simulink model "gm_soc_dvbs2_fpga"  (R2025b)
settings: Solver=VariableStepAuto  StartTime=0.0  StopTime=10.0  RelTol=1e-3
InitFcn:
  | soc_dvbs2_init;
undefined symbols (not defined in the file or in its folder): Add, coefficientsLog, coefficientsSqrt1, coefficientsSqrt2, dataBits, Deinterleaver, designMultirateFIR, noisePow, Shift, Short, soc_dvbs2_designFIRFilter, soc_dvbs2_txPacketBits, syncWord, txDataOut, txFiltCoeff, XData
libraries: simulink x304, hdlsllib x265, dspsigops x15, dsphdlfiltering2 x8, hdlmdlgenlib x6, dsphdlsigops2 x5, commseqgen3 x5, dsphdlmathfun2 x3, hwlogicconnlib x2, whdledac x2, commhdlcrc x2, whdlutilities x1
(part 33 of 36)

== system gm_soc_dvbs2_fpga/DVBS2/DVBS2 TxRx/DVB-S2 HDL Receiver/Synchronizer and PL Header Decoder/PL Header Recovery/PL Header Decoder/ML Decoder/Integer to Bit Convertor/For Each Subsystem6_instance5 ==
  note: For Each
  In1 : Inport  OutDataTypeStr=fixdt(0, 4, 0)  PortDimensions=1  SampleTime=2.5e-07
  Extract Bits2 : simulink/Logic and Bit Operations/Extract Bits  bitsToExtract=Upper half  numBits=8  bitIdxRange=[32 63]  outScalingMode=Treat bit field as an integer
  Extract Bits3 : simulink/Logic and Bit Operations/Extract Bits  bitsToExtract=Lower half  numBits=8  bitIdxRange=[32 63]  outScalingMode=Treat bit field as an integer
  Mux1 : Mux  Inputs=2
  Out1 : Outport  SampleTime=2.5e-07
  wires:
  In1/1 -> Extract Bits2/1, Extract Bits3/1
  Extract Bits3/1 -> Mux1/2
  Extract Bits2/1 -> Mux1/1
  Mux1/1 -> Out1/1

== system gm_soc_dvbs2_fpga/DVBS2/DVBS2 TxRx/DVB-S2 HDL Receiver/Synchronizer and PL Header Decoder/PL Header Recovery/PL Header Decoder/ML Decoder/Integer to Bit Convertor/For Each Subsystem6_instance6 ==
  note: For Each
  In1 : Inport  OutDataTypeStr=fixdt(0, 4, 0)  PortDimensions=1  SampleTime=2.5e-07
  Extract Bits2 : simulink/Logic and Bit Operations/Extract Bits  bitsToExtract=Upper half  numBits=8  bitIdxRange=[32 63]  outScalingMode=Treat bit field as an integer
  Extract Bits3 : simulink/Logic and Bit Operations/Extract Bits  bitsToExtract=Lower half  numBits=8  bitIdxRange=[32 63]  outScalingMode=Treat bit field as an integer
  Mux1 : Mux  Inputs=2
  Out1 : Outport  SampleTime=2.5e-07
  wires:
  Extract Bits3/1 -> Mux1/2
  In1/1 -> Extract Bits2/1, Extract Bits3/1
  Extract Bits2/1 -> Mux1/1
  Mux1/1 -> Out1/1

== system gm_soc_dvbs2_fpga/DVBS2/DVBS2 TxRx/DVB-S2 HDL Receiver/Synchronizer and PL Header Decoder/PL Header Recovery/PL Header Decoder/ML Decoder/Integer to Bit Convertor/For Each Subsystem6_instance7 ==
  note: For Each
  In1 : Inport  OutDataTypeStr=fixdt(0, 4, 0)  PortDimensions=1  SampleTime=2.5e-07
  Extract Bits2 : simulink/Logic and Bit Operations/Extract Bits  bitsToExtract=Upper half  numBits=8  bitIdxRange=[32 63]  outScalingMode=Treat bit field as an integer
  Extract Bits3 : simulink/Logic and Bit Operations/Extract Bits  bitsToExtract=Lower half  numBits=8  bitIdxRange=[32 63]  outScalingMode=Treat bit field as an integer
  Mux1 : Mux  Inputs=2
  Out1 : Outport  SampleTime=2.5e-07
  wires:
  In1/1 -> Extract Bits2/1, Extract Bits3/1
  Extract Bits3/1 -> Mux1/2
  Extract Bits2/1 -> Mux1/1
  Mux1/1 -> Out1/1

== system gm_soc_dvbs2_fpga/DVBS2/DVBS2 TxRx/DVB-S2 HDL Receiver/Synchronizer and PL Header Decoder/PL Header Recovery/PL Header Decoder/ML Decoder/Integer to Bit Convertor/For Each Subsystem6_instance8 ==
  note: For Each
  In1 : Inport  OutDataTypeStr=fixdt(0, 4, 0)  PortDimensions=1  SampleTime=2.5e-07
  Extract Bits2 : simulink/Logic and Bit Operations/Extract Bits  bitsToExtract=Upper half  numBits=8  bitIdxRange=[32 63]  outScalingMode=Treat bit field as an integer
  Extract Bits3 : simulink/Logic and Bit Operations/Extract Bits  bitsToExtract=Lower half  numBits=8  bitIdxRange=[32 63]  outScalingMode=Treat bit field as an integer
  Mux1 : Mux  Inputs=2
  Out1 : Outport  SampleTime=2.5e-07
  wires:
  In1/1 -> Extract Bits3/1, Extract Bits2/1
  Extract Bits2/1 -> Mux1/1
  Extract Bits3/1 -> Mux1/2
  Mux1/1 -> Out1/1

== system gm_soc_dvbs2_fpga/DVBS2/DVBS2 TxRx/DVB-S2 HDL Receiver/Synchronizer and PL Header Decoder/PL Header Recovery/PL Header Decoder/ML Decoder/Integer to Bit Convertor/For Each Subsystem7_instance1 ==
  note: For Each
  In1 : Inport  OutDataTypeStr=fixdt(0, 2, 0)  PortDimensions=1  SampleTime=2.5e-07
  Extract Bits2 : simulink/Logic and Bit Operations/Extract Bits  bitsToExtract=Upper half  numBits=8  bitIdxRange=[32 63]  outScalingMode=Treat bit field as an integer
  Extract Bits3 : simulink/Logic and Bit Operations/Extract Bits  bitsToExtract=Lower half  numBits=8  bitIdxRange=[32 63]  outScalingMode=Treat bit field as an integer
  Mux1 : Mux  Inputs=2
  Out1 : Outport  SampleTime=2.5e-07
  wires:
  Extract Bits3/1 -> Mux1/2
  In1/1 -> Extract Bits2/1, Extract Bits3/1
  Extract Bits2/1 -> Mux1/1
  Mux1/1 -> Out1/1

== system gm_soc_dvbs2_fpga/DVBS2/DVBS2 TxRx/DVB-S2 HDL Receiver/Synchronizer and PL Header Decoder/PL Header Recovery/PL Header Decoder/ML Decoder/Integer to Bit Convertor/For Each Subsystem7_instance10 ==
  note: For Each
  In1 : Inport  OutDataTypeStr=fixdt(0, 2, 0)  PortDimensions=1  SampleTime=2.5e-07
  Extract Bits2 : simulink/Logic and Bit Operations/Extract Bits  bitsToExtract=Upper half  numBits=8  bitIdxRange=[32 63]  outScalingMode=Treat bit field as an integer
  Extract Bits3 : simulink/Logic and Bit Operations/Extract Bits  bitsToExtract=Lower half  numBits=8  bitIdxRange=[32 63]  outScalingMode=Treat bit field as an integer
  Mux1 : Mux  Inputs=2
  Out1 : Outport  SampleTime=2.5e-07
  wires:
  In1/1 -> Extract Bits2/1, Extract Bits3/1
  Extract Bits3/1 -> Mux1/2
  Extract Bits2/1 -> Mux1/1
  Mux1/1 -> Out1/1

== system gm_soc_dvbs2_fpga/DVBS2/DVBS2 TxRx/DVB-S2 HDL Receiver/Synchronizer and PL Header Decoder/PL Header Recovery/PL Header Decoder/ML Decoder/Integer to Bit Convertor/For Each Subsystem7_instance11 ==
  note: For Each
  In1 : Inport  OutDataTypeStr=fixdt(0, 2, 0)  PortDimensions=1  SampleTime=2.5e-07
  Extract Bits2 : simulink/Logic and Bit Operations/Extract Bits  bitsToExtract=Upper half  numBits=8  bitIdxRange=[32 63]  outScalingMode=Treat bit field as an integer
  Extract Bits3 : simulink/Logic and Bit Operations/Extract Bits  bitsToExtract=Lower half  numBits=8  bitIdxRange=[32 63]  outScalingMode=Treat bit field as an integer
  Mux1 : Mux  Inputs=2
  Out1 : Outport  SampleTime=2.5e-07
  wires:
  In1/1 -> Extract Bits2/1, Extract Bits3/1
  Extract Bits2/1 -> Mux1/1
  Extract Bits3/1 -> Mux1/2
  Mux1/1 -> Out1/1

== system gm_soc_dvbs2_fpga/DVBS2/DVBS2 TxRx/DVB-S2 HDL Receiver/Synchronizer and PL Header Decoder/PL Header Recovery/PL Header Decoder/ML Decoder/Integer to Bit Convertor/For Each Subsystem7_instance12 ==
  note: For Each
  In1 : Inport  OutDataTypeStr=fixdt(0, 2, 0)  PortDimensions=1  SampleTime=2.5e-07
  Extract Bits2 : simulink/Logic and Bit Operations/Extract Bits  bitsToExtract=Upper half  numBits=8  bitIdxRange=[32 63]  outScalingMode=Treat bit field as an integer
  Extract Bits3 : simulink/Logic and Bit Operations/Extract Bits  bitsToExtract=Lower half  numBits=8  bitIdxRange=[32 63]  outScalingMode=Treat bit field as an integer
  Mux1 : Mux  Inputs=2
  Out1 : Outport  SampleTime=2.5e-07
  wires:
  Extract Bits3/1 -> Mux1/2
  In1/1 -> Extract Bits2/1, Extract Bits3/1
  Extract Bits2/1 -> Mux1/1
  Mux1/1 -> Out1/1

== system gm_soc_dvbs2_fpga/DVBS2/DVBS2 TxRx/DVB-S2 HDL Receiver/Synchronizer and PL Header Decoder/PL Header Recovery/PL Header Decoder/ML Decoder/Integer to Bit Convertor/For Each Subsystem7_instance13 ==
  note: For Each
  In1 : Inport  OutDataTypeStr=fixdt(0, 2, 0)  PortDimensions=1  SampleTime=2.5e-07
  Extract Bits2 : simulink/Logic and Bit Operations/Extract Bits  bitsToExtract=Upper half  numBits=8  bitIdxRange=[32 63]  outScalingMode=Treat bit field as an integer
  Extract Bits3 : simulink/Logic and Bit Operations/Extract Bits  bitsToExtract=Lower half  numBits=8  bitIdxRange=[32 63]  outScalingMode=Treat bit field as an integer
  Mux1 : Mux  Inputs=2
  Out1 : Outport  SampleTime=2.5e-07
  wires:
  In1/1 -> Extract Bits2/1, Extract Bits3/1
  Extract Bits3/1 -> Mux1/2
  Extract Bits2/1 -> Mux1/1
  Mux1/1 -> Out1/1

== system gm_soc_dvbs2_fpga/DVBS2/DVBS2 TxRx/DVB-S2 HDL Receiver/Synchronizer and PL Header Decoder/PL Header Recovery/PL Header Decoder/ML Decoder/Integer to Bit Convertor/For Each Subsystem7_instance14 ==
  note: For Each
  In1 : Inport  OutDataTypeStr=fixdt(0, 2, 0)  PortDimensions=1  SampleTime=2.5e-07
  Extract Bits2 : simulink/Logic and Bit Operations/Extract Bits  bitsToExtract=Upper half  numBits=8  bitIdxRange=[32 63]  outScalingMode=Treat bit field as an integer
  Extract Bits3 : simulink/Logic and Bit Operations/Extract Bits  bitsToExtract=Lower half  numBits=8  bitIdxRange=[32 63]  outScalingMode=Treat bit field as an integer
  Mux1 : Mux  Inputs=2
  Out1 : Outport  SampleTime=2.5e-07
  wires:
  Extract Bits3/1 -> Mux1/2
  In1/1 -> Extract Bits2/1, Extract Bits3/1
  Extract Bits2/1 -> Mux1/1
  Mux1/1 -> Out1/1

== system gm_soc_dvbs2_fpga/DVBS2/DVBS2 TxRx/DVB-S2 HDL Receiver/Synchronizer and PL Header Decoder/PL Header Recovery/PL Header Decoder/ML Decoder/Integer to Bit Convertor/For Each Subsystem7_instance15 ==
  note: For Each
  In1 : Inport  OutDataTypeStr=fixdt(0, 2, 0)  PortDimensions=1  SampleTime=2.5e-07
  Extract Bits2 : simulink/Logic and Bit Operations/Extract Bits  bitsToExtract=Upper half  numBits=8  bitIdxRange=[32 63]  outScalingMode=Treat bit field as an integer
  Extract Bits3 : simulink/Logic and Bit Operations/Extract Bits  bitsToExtract=Lower half  numBits=8  bitIdxRange=[32 63]  outScalingMode=Treat bit field as an integer
  Mux1 : Mux  Inputs=2
  Out1 : Outport  SampleTime=2.5e-07
  wires:
  In1/1 -> Extract Bits2/1, Extract Bits3/1
  Extract Bits3/1 -> Mux1/2
  Extract Bits2/1 -> Mux1/1
  Mux1/1 -> Out1/1

== system gm_soc_dvbs2_fpga/DVBS2/DVBS2 TxRx/DVB-S2 HDL Receiver/Synchronizer and PL Header Decoder/PL Header Recovery/PL Header Decoder/ML Decoder/Integer to Bit Convertor/For Each Subsystem7_instance16 ==
  note: For Each
  In1 : Inport  OutDataTypeStr=fixdt(0, 2, 0)  PortDimensions=1  SampleTime=2.5e-07
  Extract Bits2 : simulink/Logic and Bit Operations/Extract Bits  bitsToExtract=Upper half  numBits=8  bitIdxRange=[32 63]  outScalingMode=Treat bit field as an integer
  Extract Bits3 : simulink/Logic and Bit Operations/Extract Bits  bitsToExtract=Lower half  numBits=8  bitIdxRange=[32 63]  outScalingMode=Treat bit field as an integer
  Mux1 : Mux  Inputs=2
  Out1 : Outport  SampleTime=2.5e-07
  wires:
  Extract Bits3/1 -> Mux1/2
  In1/1 -> Extract Bits2/1, Extract Bits3/1
  Extract Bits2/1 -> Mux1/1
  Mux1/1 -> Out1/1

== system gm_soc_dvbs2_fpga/DVBS2/DVBS2 TxRx/DVB-S2 HDL Receiver/Synchronizer and PL Header Decoder/PL Header Recovery/PL Header Decoder/ML Decoder/Integer to Bit Convertor/For Each Subsystem7_instance2 ==
  note: For Each
  In1 : Inport  OutDataTypeStr=fixdt(0, 2, 0)  PortDimensions=1  SampleTime=2.5e-07
  Extract Bits2 : simulink/Logic and Bit Operations/Extract Bits  bitsToExtract=Upper half  numBits=8  bitIdxRange=[32 63]  outScalingMode=Treat bit field as an integer
  Extract Bits3 : simulink/Logic and Bit Operations/Extract Bits  bitsToExtract=Lower half  numBits=8  bitIdxRange=[32 63]  outScalingMode=Treat bit field as an integer
  Mux1 : Mux  Inputs=2
  Out1 : Outport  SampleTime=2.5e-07
  wires:
  Extract Bits3/1 -> Mux1/2
  In1/1 -> Extract Bits2/1, Extract Bits3/1
  Extract Bits2/1 -> Mux1/1
  Mux1/1 -> Out1/1

== system gm_soc_dvbs2_fpga/DVBS2/DVBS2 TxRx/DVB-S2 HDL Receiver/Synchronizer and PL Header Decoder/PL Header Recovery/PL Header Decoder/ML Decoder/Integer to Bit Convertor/For Each Subsystem7_instance3 ==
  note: For Each
  In1 : Inport  OutDataTypeStr=fixdt(0, 2, 0)  PortDimensions=1  SampleTime=2.5e-07
  Extract Bits2 : simulink/Logic and Bit Operations/Extract Bits  bitsToExtract=Upper half  numBits=8  bitIdxRange=[32 63]  outScalingMode=Treat bit field as an integer
  Extract Bits3 : simulink/Logic and Bit Operations/Extract Bits  bitsToExtract=Lower half  numBits=8  bitIdxRange=[32 63]  outScalingMode=Treat bit field as an integer
  Mux1 : Mux  Inputs=2
  Out1 : Outport  SampleTime=2.5e-07
  wires:
  In1/1 -> Extract Bits2/1, Extract Bits3/1
  Extract Bits3/1 -> Mux1/2
  Extract Bits2/1 -> Mux1/1
  Mux1/1 -> Out1/1

== system gm_soc_dvbs2_fpga/DVBS2/DVBS2 TxRx/DVB-S2 HDL Receiver/Synchronizer and PL Header Decoder/PL Header Recovery/PL Header Decoder/ML Decoder/Integer to Bit Convertor/For Each Subsystem7_instance4 ==
  note: For Each
  In1 : Inport  OutDataTypeStr=fixdt(0, 2, 0)  PortDimensions=1  SampleTime=2.5e-07
  Extract Bits2 : simulink/Logic and Bit Operations/Extract Bits  bitsToExtract=Upper half  numBits=8  bitIdxRange=[32 63]  outScalingMode=Treat bit field as an integer
  Extract Bits3 : simulink/Logic and Bit Operations/Extract Bits  bitsToExtract=Lower half  numBits=8  bitIdxRange=[32 63]  outScalingMode=Treat bit field as an integer
  Mux1 : Mux  Inputs=2
  Out1 : Outport  SampleTime=2.5e-07
  wires:
  Extract Bits3/1 -> Mux1/2
  In1/1 -> Extract Bits2/1, Extract Bits3/1
  Extract Bits2/1 -> Mux1/1
  Mux1/1 -> Out1/1

== system gm_soc_dvbs2_fpga/DVBS2/DVBS2 TxRx/DVB-S2 HDL Receiver/Synchronizer and PL Header Decoder/PL Header Recovery/PL Header Decoder/ML Decoder/Integer to Bit Convertor/For Each Subsystem7_instance5 ==
  note: For Each
  In1 : Inport  OutDataTypeStr=fixdt(0, 2, 0)  PortDimensions=1  SampleTime=2.5e-07
  Extract Bits2 : simulink/Logic and Bit Operations/Extract Bits  bitsToExtract=Upper half  numBits=8  bitIdxRange=[32 63]  outScalingMode=Treat bit field as an integer
  Extract Bits3 : simulink/Logic and Bit Operations/Extract Bits  bitsToExtract=Lower half  numBits=8  bitIdxRange=[32 63]  outScalingMode=Treat bit field as an integer
  Mux1 : Mux  Inputs=2
  Out1 : Outport  SampleTime=2.5e-07
  wires:
  In1/1 -> Extract Bits2/1, Extract Bits3/1
  Extract Bits3/1 -> Mux1/2
  Extract Bits2/1 -> Mux1/1
  Mux1/1 -> Out1/1

== system gm_soc_dvbs2_fpga/DVBS2/DVBS2 TxRx/DVB-S2 HDL Receiver/Synchronizer and PL Header Decoder/PL Header Recovery/PL Header Decoder/ML Decoder/Integer to Bit Convertor/For Each Subsystem7_instance6 ==
  note: For Each
  In1 : Inport  OutDataTypeStr=fixdt(0, 2, 0)  PortDimensions=1  SampleTime=2.5e-07
  Extract Bits2 : simulink/Logic and Bit Operations/Extract Bits  bitsToExtract=Upper half  numBits=8  bitIdxRange=[32 63]  outScalingMode=Treat bit field as an integer
  Extract Bits3 : simulink/Logic and Bit Operations/Extract Bits  bitsToExtract=Lower half  numBits=8  bitIdxRange=[32 63]  outScalingMode=Treat bit field as an integer
  Mux1 : Mux  Inputs=2
  Out1 : Outport  SampleTime=2.5e-07
  wires:
  In1/1 -> Extract Bits2/1, Extract Bits3/1
  Extract Bits2/1 -> Mux1/1
  Extract Bits3/1 -> Mux1/2
  Mux1/1 -> Out1/1

== system gm_soc_dvbs2_fpga/DVBS2/DVBS2 TxRx/DVB-S2 HDL Receiver/Synchronizer and PL Header Decoder/PL Header Recovery/PL Header Decoder/ML Decoder/Integer to Bit Convertor/For Each Subsystem7_instance7 ==
  note: For Each
  In1 : Inport  OutDataTypeStr=fixdt(0, 2, 0)  PortDimensions=1  SampleTime=2.5e-07
  Extract Bits2 : simulink/Logic and Bit Operations/Extract Bits  bitsToExtract=Upper half  numBits=8  bitIdxRange=[32 63]  outScalingMode=Treat bit field as an integer
  Extract Bits3 : simulink/Logic and Bit Operations/Extract Bits  bitsToExtract=Lower half  numBits=8  bitIdxRange=[32 63]  outScalingMode=Treat bit field as an integer
  Mux1 : Mux  Inputs=2
  Out1 : Outport  SampleTime=2.5e-07
  wires:
  Extract Bits3/1 -> Mux1/2
  In1/1 -> Extract Bits2/1, Extract Bits3/1
  Extract Bits2/1 -> Mux1/1
  Mux1/1 -> Out1/1

== system gm_soc_dvbs2_fpga/DVBS2/DVBS2 TxRx/DVB-S2 HDL Receiver/Synchronizer and PL Header Decoder/PL Header Recovery/PL Header Decoder/ML Decoder/Integer to Bit Convertor/For Each Subsystem7_instance8 ==
  note: For Each
  In1 : Inport  OutDataTypeStr=fixdt(0, 2, 0)  PortDimensions=1  SampleTime=2.5e-07
  Extract Bits2 : simulink/Logic and Bit Operations/Extract Bits  bitsToExtract=Upper half  numBits=8  bitIdxRange=[32 63]  outScalingMode=Treat bit field as an integer
  Extract Bits3 : simulink/Logic and Bit Operations/Extract Bits  bitsToExtract=Lower half  numBits=8  bitIdxRange=[32 63]  outScalingMode=Treat bit field as an integer
  Mux1 : Mux  Inputs=2
  Out1 : Outport  SampleTime=2.5e-07
  wires:
  In1/1 -> Extract Bits3/1, Extract Bits2/1
  Extract Bits3/1 -> Mux1/2
  Extract Bits2/1 -> Mux1/1
  Mux1/1 -> Out1/1

== system gm_soc_dvbs2_fpga/DVBS2/DVBS2 TxRx/DVB-S2 HDL Receiver/Synchronizer and PL Header Decoder/PL Header Recovery/PL Header Decoder/ML Decoder/Integer to Bit Convertor/For Each Subsystem7_instance9 ==
  note: For Each
  In1 : Inport  OutDataTypeStr=fixdt(0, 2, 0)  PortDimensions=1  SampleTime=2.5e-07
  Extract Bits2 : simulink/Logic and Bit Operations/Extract Bits  bitsToExtract=Upper half  numBits=8  bitIdxRange=[32 63]  outScalingMode=Treat bit field as an integer
  Extract Bits3 : simulink/Logic and Bit Operations/Extract Bits  bitsToExtract=Lower half  numBits=8  bitIdxRange=[32 63]  outScalingMode=Treat bit field as an integer
  Mux1 : Mux  Inputs=2
  Out1 : Outport  SampleTime=2.5e-07
  wires:
  Extract Bits3/1 -> Mux1/2
  In1/1 -> Extract Bits2/1, Extract Bits3/1
  Extract Bits2/1 -> Mux1/1
  Mux1/1 -> Out1/1

== system gm_soc_dvbs2_fpga/DVBS2/DVBS2 TxRx/DVB-S2 HDL Receiver/Synchronizer and PL Header Decoder/PL Header Recovery/PL Header Decoder/ML Decoder/Integer to Bit Convertor/For Each Subsystem_instance1 ==
  note: For Each
  In1 : Inport  OutDataTypeStr=uint16  PortDimensions=1  SampleTime=2.5e-07
  Extract Bits2 : simulink/Logic and Bit Operations/Extract Bits  bitsToExtract=Upper half  numBits=8  bitIdxRange=[32 63]  outScalingMode=Treat bit field as an integer
  Extract Bits3 : simulink/Logic and Bit Operations/Extract Bits  bitsToExtract=Lower half  numBits=8  bitIdxRange=[32 63]  outScalingMode=Treat bit field as an integer
  Mux1 : Mux  Inputs=2
  Out1 : Outport  SampleTime=2.5e-07
  wires:
  In1/1 -> Extract Bits2/1, Extract Bits3/1
  Extract Bits3/1 -> Mux1/2
  Extract Bits2/1 -> Mux1/1
  Mux1/1 -> Out1/1

== system gm_soc_dvbs2_fpga/DVBS2/DVBS2 TxRx/DVB-S2 HDL Receiver/Synchronizer and PL Header Decoder/PL Header Recovery/PL Header Decoder/ML Decoder/Integer to Bit Convertor/For Each Subsystem_instance2 ==
  note: For Each
  In1 : Inport  OutDataTypeStr=uint16  PortDimensions=1  SampleTime=2.5e-07
  Extract Bits2 : simulink/Logic and Bit Operations/Extract Bits  bitsToExtract=Upper half  numBits=8  bitIdxRange=[32 63]  outScalingMode=Treat bit field as an integer
  Extract Bits3 : simulink/Logic and Bit Operations/Extract Bits  bitsToExtract=Lower half  numBits=8  bitIdxRange=[32 63]  outScalingMode=Treat bit field as an integer
  Mux1 : Mux  Inputs=2
  Out1 : Outport  SampleTime=2.5e-07
  wires:
  In1/1 -> Extract Bits2/1, Extract Bits3/1
  Extract Bits2/1 -> Mux1/1
  Extract Bits3/1 -> Mux1/2
  Mux1/1 -> Out1/1

== system gm_soc_dvbs2_fpga/DVBS2/DVBS2 TxRx/DVB-S2 HDL Receiver/Synchronizer and PL Header Decoder/PL Header Recovery/PL Header Decoder/ML Decoder/Integer to Bit Convertor/Subsystem ==
  u : Inport  OutDataTypeStr=uint32  PortDimensions=1  SampleTime=2.5e-07
  u1 : Inport  Port=2  OutDataTypeStr=uint32  PortDimensions=1  SampleTime=2.5e-07
  Extract Bits2 : simulink/Logic and Bit Operations/Extract Bits  bitsToExtract=Upper half  numBits=8  bitIdxRange=[32 63]  outScalingMode=Treat bit field as an integer
  Extract Bits3 : simulink/Logic and Bit Operations/Extract Bits  bitsToExtract=Lower half  numBits=8  bitIdxRange=[32 63]  outScalingMode=Treat bit field as an integer
  Mux1 : Mux  Inputs=2
  Out1 : Outport  SampleTime=2.5e-07
  wires:
  u/1 -> Extract Bits2/1
  u1/1 -> Extract Bits3/1
  Extract Bits3/1 -> Mux1/2
  Extract Bits2/1 -> Mux1/1
  Mux1/1 -> Out1/1

== system gm_soc_dvbs2_fpga/DVBS2/DVBS2 TxRx/DVB-S2 HDL Receiver/Synchronizer and PL Header Decoder/PL Header Recovery/PL Header Decoder/ML Decoder/Integer to Bit Convertor/Subsystem1 ==
  u : Inport  OutDataTypeStr=uint32  PortDimensions=1  SampleTime=2.5e-07
  u1 : Inport  Port=2  OutDataTypeStr=uint32  PortDimensions=1  SampleTime=2.5e-07
  Extract Bits2 : simulink/Logic and Bit Operations/Extract Bits  bitsToExtract=Upper half  numBits=8  bitIdxRange=[32 63]  outScalingMode=Treat bit field as an integer
  Extract Bits3 : simulink/Logic and Bit Operations/Extract Bits  bitsToExtract=Lower half  numBits=8  bitIdxRange=[32 63]  outScalingMode=Treat bit field as an integer
  Mux1 : Mux  Inputs=2
  Out1 : Outport  SampleTime=2.5e-07
  wires:
  u1/1 -> Extract Bits3/1
  u/1 -> Extract Bits2/1
  Extract Bits2/1 -> Mux1/1
  Extract Bits3/1 -> Mux1/2
  Mux1/1 -> Out1/1

== system gm_soc_dvbs2_fpga/DVBS2/DVBS2 TxRx/DVB-S2 HDL Receiver/Synchronizer and PL Header Decoder/Time Frequency and Coarse Phase Synchronizer/Coarse Phase Synchronizer/Coarse Phase Corrector/Reciprocal/Function Impl ==
  switch : Inport  OutDataTypeStr=fixdt(0, 1, 0)  PortDimensions=1  SampleTime=2.5e-07
  LUTAddr : Inport  Port=2  OutDataTypeStr=fixdt(0, 12, 0)  PortDimensions=1  SampleTime=2.5e-07
  Delay{6..8,10,15..16} (6 alike) : Delay
  Delay9 : Delay  DelayLength=1
  LUT1 : LookupNDDirect  NumberOfTableDimensions=1  Table=LUT(:,1)  DiagnosticForOutOfRangeInput=Error
  LUT2 : LookupNDDirect  NumberOfTableDimensions=1  Table=LUT(:,2)  DiagnosticForOutOfRangeInput=Error
  Multiport Switch : MultiPortSwitch  DataPortOrder=Zero-based contiguous  Inputs=2  zeroidx=on  OutDataTypeStr=fixdt(1, 26, 14)  SaturateOnIntegerOverflow=off  InputSameDT=off
  functionValues : Outport  SampleTime=2.5e-07
  wires:
  LUT1/1 -> Delay16/1
  Delay8/1 -> Delay10/1
  LUTAddr/1 -> Delay7/1, Delay6/1
  Delay6/1 -> LUT1/1
  Delay10/1 -> Multiport Switch/1
  LUT2/1 -> Delay15/1
  Delay7/1 -> LUT2/1
  Delay16/1 -> Multiport Switch/3
  switch/1 -> Delay8/1
  Delay15/1 -> Multiport Switch/2
  Multiport Switch/1 -> Delay9/1
  Delay9/1 -> functionValues/1

== system gm_soc_dvbs2_fpga/DVBS2/DVBS2 TxRx/DVB-S2 HDL Receiver/Synchronizer and PL Header Decoder/Time Frequency and Coarse Phase Synchronizer/Fine Frequency Synchronizer/Modified L and R Algorithm/L and R Algorithm 18 point/Compute R(m) for 1 to 6 ==
  z : Inport  OutDataTypeStr=fixdt(1, 16, 11)  PortDimensions=1  SampleTime=2.5e-07
      settings: SignalType=complex
  zvalid : Inport  Port=2  OutDataTypeStr=boolean  PortDimensions=1  SampleTime=2.5e-07
  Add2 : Sum  Inputs=++++++  OutDataTypeStr=fixdt(1, 36, 22)
  Compute R(m)_1 : Subsystem  mask{m=double(1), N=double(36)}
      mask prompts: m "m value :"; N "N value :"
      mask init:
      | MulDivFactor = fi(0,0,16,21,"hex","ea0f");
      | N = double(36);
      | m = double(1);
  Compute R(m)_2 : Subsystem  mask{m=double(2), N=double(36)}
      mask prompts: m "m value :"; N "N value :"
      mask init:
      | MulDivFactor = fi(0,0,16,21,"hex","f0f1");
      | N = double(36);
      | m = double(2);
  Compute R(m)_3 : Subsystem  mask{m=double(3), N=double(36)}
      mask prompts: m "m value :"; N "N value :"
      mask init:
      | MulDivFactor = fi(0,0,16,21,"hex","f83e");
      | N = double(36);
      | m = double(3);
  Compute R(m)_4 : Subsystem  mask{m=double(4), N=double(36)}
      mask prompts: m "m value :"; N "N value :"
      mask init:
      | MulDivFactor = fi(0,0,16,20,"hex","8000");
      | N = double(36);
      | m = double(4);
  Compute R(m)_5 : Subsystem  mask{m=double(5), N=double(36)}
      mask prompts: m "m value :"; N "N value :"
      mask init:
      | MulDivFactor = fi(0,0,16,20,"hex","8421");
      | N = double(36);
      | m = double(5);
  Compute R(m)_6 : Subsystem  mask{m=double(6), N=double(36)}
      mask prompts: m "m value :"; N "N value :"
      mask init:
      | MulDivFactor = fi(0,0,16,20,"hex","8889");
      | N = double(36);
      | m = double(6);
  Delay{1..7} (7 alike) : Delay
  sum : Outport  SampleTime=2.5e-07
  wires:
  Compute R(m)_3/1(Out1) -> Delay2/1
  z/1 -> Compute R(m)_6/1(z), Compute R(m)_5/1(z), Compute R(m)_4/1(z), Compute R(m)_2/1(z), Compute R(m)_3/1(z), Compute R(m)_1/1(z)
  Compute R(m)_5/1(Out1) -> Delay5/1
  Compute R(m)_2/1(Out1) -> Delay1/1
  Compute R(m)_1/1(Out1) -> Delay3/1
  zvalid/1 -> Compute R(m)_5/2(zvalid), Compute R(m)_4/2(zvalid), Compute R(m)_6/2(zvalid), Compute R(m)_3/2(zvalid), Compute R(m)_1/2(zvalid), Compute R(m)_2/2(zvalid)
  Compute R(m)_4/1(Out1) -> Delay4/1
  Delay1/1 -> Add2/2
  Compute R(m)_6/1(Out1) -> Delay6/1
  Delay3/1 -> Add2/1
  Delay2/1 -> Add2/3
  Delay4/1 -> Add2/4
  Delay5/1 -> Add2/5
  Delay6/1 -> Add2/6
  Add2/1 -> Delay7/1
  Delay7/1 -> sum/1

== system gm_soc_dvbs2_fpga/DVBS2/DVBS2 TxRx/DVB-S2 HDL Receiver/Synchronizer and PL Header Decoder/Time Frequency and Coarse Phase Synchronizer/Fine Frequency Synchronizer/Modified L and R Algorithm/L and R Algorithm 18 point/Compute R(m) for 13 to 18 ==
  z : Inport  OutDataTypeStr=fixdt(1, 16, 11)  PortDimensions=1  SampleTime=2.5e-07
      settings: SignalType=complex
  zvalid : Inport  Port=2  OutDataTypeStr=boolean  PortDimensions=1  SampleTime=2.5e-07
  Add2 : Sum  Inputs=++++++  OutDataTypeStr=fixdt(1, 36, 22)
  Compute R(m)_1 : Subsystem  mask{m=double(13), N=double(36)}
      mask prompts: m "m value :"; N "N value :"
      mask init:
      | MulDivFactor = fi(0,0,16,20,"hex","b216");
      | N = double(36);
      | m = double(13);
  Compute R(m)_2 : Subsystem  mask{m=double(14), N=double(36)}
      mask prompts: m "m value :"; N "N value :"
      mask init:
      | MulDivFactor = fi(0,0,16,20,"hex","ba2f");
      | N = double(36);
      | m = double(14);
  Compute R(m)_3 : Subsystem  mask{m=double(15), N=double(36)}
      mask prompts: m "m value :"; N "N value :"
      mask init:
      | MulDivFactor = fi(0,0,16,20,"hex","c30c");
      | N = double(36);
      | m = double(15);
  Compute R(m)_4 : Subsystem  mask{m=double(16), N=double(36)}
      mask prompts: m "m value :"; N "N value :"
      mask init:
      | MulDivFactor = fi(0,0,16,20,"hex","cccd");
      | N = double(36);
      | m = double(16);
  Compute R(m)_5 : Subsystem  mask{m=double(17), N=double(36)}
      mask prompts: m "m value :"; N "N value :"
      mask init:
      | MulDivFactor = fi(0,0,16,20,"hex","d794");
      | N = double(36);
      | m = double(17);
  Compute R(m)_6 : Subsystem  mask{m=double(18), N=double(36)}
      mask prompts: m "m value :"; N "N value :"
      mask init:
      | MulDivFactor = fi(0,0,16,20,"hex","e38e");
      | N = double(36);
      | m = double(18);
  Delay{1..7} (7 alike) : Delay
  sum : Outport  SampleTime=2.5e-07
  wires:
  z/1 -> Compute R(m)_5/1(z), Compute R(m)_1/1(z), Compute R(m)_4/1(z), Compute R(m)_3/1(z), Compute R(m)_6/1(z), Compute R(m)_2/1(z)
  Compute R(m)_1/1(Out1) -> Delay3/1
  Delay5/1 -> Add2/5
  zvalid/1 -> Compute R(m)_5/2(zvalid), Compute R(m)_6/2(zvalid), Compute R(m)_3/2(zvalid), Compute R(m)_4/2(zvalid), Compute R(m)_1/2(zvalid), Compute R(m)_2/2(zvalid)
  Compute R(m)_2/1(Out1) -> Delay1/1
  Compute R(m)_3/1(Out1) -> Delay2/1
  Compute R(m)_6/1(Out1) -> Delay6/1
  Compute R(m)_4/1(Out1) -> Delay4/1
  Compute R(m)_5/1(Out1) -> Delay5/1
  Delay3/1 -> Add2/1
  Delay1/1 -> Add2/2
  Delay2/1 -> Add2/3
  Delay4/1 -> Add2/4
  Delay6/1 -> Add2/6
  Add2/1 -> Delay7/1
  Delay7/1 -> sum/1

== system gm_soc_dvbs2_fpga/DVBS2/DVBS2 TxRx/DVB-S2 HDL Receiver/Synchronizer and PL Header Decoder/Time Frequency and Coarse Phase Synchronizer/Fine Frequency Synchronizer/Modified L and R Algorithm/L and R Algorithm 18 point/Compute R(m) for 7 to 12 ==
  z : Inport  OutDataTypeStr=fixdt(1, 16, 11)  PortDimensions=1  SampleTime=2.5e-07
      settings: SignalType=complex
  zvalid : Inport  Port=2  OutDataTypeStr=boolean  PortDimensions=1  SampleTime=2.5e-07
  Add2 : Sum  Inputs=++++++  OutDataTypeStr=fixdt(1, 36, 22)
  Compute R(m)_1 : Subsystem  mask{m=double(7), N=double(36)}
      mask prompts: m "m value :"; N "N value :"
      mask init:
      | MulDivFactor = fi(0,0,16,20,"hex","8d3e");
      | N = double(36);
      | m = double(7);
  Compute R(m)_2 : Subsystem  mask{m=double(8), N=double(36)}
      mask prompts: m "m value :"; N "N value :"
      mask init:
      | MulDivFactor = fi(0,0,16,20,"hex","9249");
      | N = double(36);
      | m = double(8);
  Compute R(m)_3 : Subsystem  mask{m=double(9), N=double(36)}
      mask prompts: m "m value :"; N "N value :"
      mask init:
      | MulDivFactor = fi(0,0,16,20,"hex","97b4");
      | N = double(36);
      | m = double(9);
  Compute R(m)_4 : Subsystem  mask{m=double(10), N=double(36)}
      mask prompts: m "m value :"; N "N value :"
      mask init:
      | MulDivFactor = fi(0,0,16,20,"hex","9d8a");
      | N = double(36);
      | m = double(10);
  Compute R(m)_5 : Subsystem  mask{m=double(11), N=double(36)}
      mask prompts: m "m value :"; N "N value :"
      mask init:
      | MulDivFactor = fi(0,0,16,20,"hex","a3d7");
      | N = double(36);
      | m = double(11);
  Compute R(m)_6 : Subsystem  mask{m=double(12), N=double(36)}
      mask prompts: m "m value :"; N "N value :"
      mask init:
      | MulDivFactor = fi(0,0,16,20,"hex","aaab");
      | N = double(36);
      | m = double(12);
  Delay{1..7} (7 alike) : Delay
  sum : Outport  SampleTime=2.5e-07
  wires:
  Compute R(m)_2/1(Out1) -> Delay1/1
  z/1 -> Compute R(m)_4/1(z), Compute R(m)_2/1(z), Compute R(m)_6/1(z), Compute R(m)_3/1(z), Compute R(m)_1/1(z), Compute R(m)_5/1(z)
  Compute R(m)_1/1(Out1) -> Delay3/1
  zvalid/1 -> Compute R(m)_4/2(zvalid), Compute R(m)_3/2(zvalid), Compute R(m)_2/2(zvalid), Compute R(m)_6/2(zvalid), Compute R(m)_5/2(zvalid), Compute R(m)_1/2(zvalid)
  Compute R(m)_3/1(Out1) -> Delay2/1
  Compute R(m)_4/1(Out1) -> Delay4/1
  Compute R(m)_5/1(Out1) -> Delay5/1
  Delay1/1 -> Add2/2
  Compute R(m)_6/1(Out1) -> Delay6/1
  Delay3/1 -> Add2/1
  Delay2/1 -> Add2/3
  Delay4/1 -> Add2/4
  Delay5/1 -> Add2/5
  Delay6/1 -> Add2/6
  Add2/1 -> Delay7/1
  Delay7/1 -> sum/1

== system gm_soc_dvbs2_fpga/DVBS2/DVBS2 TxRx/DVB-S2 HDL Receiver/Synchronizer and PL Header Decoder/Time Frequency and Coarse Phase Synchronizer/Time and Coarse Frequency Synchronizer/Coarse Frequency Estimator/Frequency Error Detector/Complex Multiplier ==
  In1 : Inport  OutDataTypeStr=fixdt(1, 18, 13)  PortDimensions=1  SampleTime=2.5e-07
      settings: SignalType=complex
  In2 : Inport  Port=2  OutDataTypeStr=fixdt(1, 18, 13)  PortDimensions=1  SampleTime=2.5e-07
      settings: SignalType=complex
  AddADn : Sum  Inputs=++|  OutDataTypeStr=fixdt(1, 37, 26)
  AddAUp : Sum  Inputs=|+-  OutDataTypeStr=fixdt(1, 37, 26)
  AddBCtr : Sum  Inputs=+|+  OutDataTypeStr=fixdt(1, 19, 13)
  AddBDn : Sum  Inputs=|+-  OutDataTypeStr=fixdt(1, 19, 13)
  AddBUp : Sum  Inputs=++|  OutDataTypeStr=fixdt(1, 19, 13)
  Complex to Real-Imag : ComplexToRealImag
  Complex to Real-Imag1 : ComplexToRealImag
  Delay{1..5,8..20} (18 alike) : Delay  DelayLength=1
  Delay{6..7,21..27} (9 alike) : Delay
  Product : Product  OutDataTypeStr=fixdt(1, 37, 26)
  Product1 : Product  OutDataTypeStr=fixdt(1, 37, 26)
  Product2 : Product  OutDataTypeStr=fixdt(1, 37, 26)
  Real-Imag to Complex : RealImagToComplex
  Out1 : Outport  SampleTime=2.5e-07  VectorParamsAs1DForOutWhenUnconnected=off
  wires:
  Delay9/1 -> AddBUp/1
  Product2/1 -> Delay27/1
  Delay7/1 -> Product/2
  [IM2] -> Delay15/1
  [RE2] -> Delay14/1
  Delay5/1 -> Delay24/1
  [IM2] -> Delay10/1
  AddAUp/1 -> Delay19/1
  Product/1 -> Delay25/1
  [RE2] -> Delay9/1
  In1/1 -> Complex to Real-Imag/1
  Delay25/1 -> Delay16/1
  Delay10/1 -> AddBUp/2
  Delay12/1 -> Delay3/1
  In2/1 -> Complex to Real-Imag1/1
  Complex to Real-Imag/1 -> Delay11/1
  Complex to Real-Imag/2 -> Delay13/1
  Complex to Real-Imag1/1 -> [RE2]
  Complex to Real-Imag1/2 -> [IM2]
  Delay14/1 -> AddBDn/1
  Delay15/1 -> AddBDn/2
  AddBUp/1 -> Delay8/1
  Delay26/1 -> Delay17/1
  Delay11/1 -> AddBCtr/1, Delay1/1
  Product1/1 -> Delay26/1
  AddBCtr/1 -> Delay2/1
  [IM2] -> Delay12/1
  Delay13/1 -> AddBCtr/2, Delay4/1
  Real-Imag to Complex/1 -> Out1/1
  AddBDn/1 -> Delay5/1
  Delay8/1 -> Delay6/1
  Delay24/1 -> Product2/2
  Delay1/1 -> Delay7/1
  Delay4/1 -> Delay23/1
  Delay6/1 -> Product/1
  Delay2/1 -> Delay21/1
  AddADn/1 -> Delay20/1
  Delay3/1 -> Delay22/1
  Delay23/1 -> Product2/1
  Delay21/1 -> Product1/1
  Delay22/1 -> Product1/2
  Delay27/1 -> Delay18/1
  Delay16/1 -> AddAUp/1
  Delay17/1 -> AddAUp/2, AddADn/1
  Delay18/1 -> AddADn/2
  Delay19/1 -> Real-Imag to Complex/1
  Delay20/1 -> Real-Imag to Complex/2

== system gm_soc_dvbs2_fpga/DVBS2/DVBS2 TxRx/DVB-S2 HDL Receiver/Synchronizer and PL Header Decoder/Time Frequency and Coarse Phase Synchronizer/Time and Coarse Frequency Synchronizer/Frame Synchronizer/Correlator/Moving Sum ==
  scaled1 : Inport  OutDataTypeStr=fixdt(1, 32, 30)  PortDimensions=1  SampleTime=2.5e-07
  scaled2 : Inport  Port=2  OutDataTypeStr=fixdt(1, 32, 30)  PortDimensions=1  SampleTime=2.5e-07
  validIn : Inport  Port=3  OutDataTypeStr=boolean  PortDimensions=1  SampleTime=2.5e-07
  Add : Sum  Inputs=+-  OutDataTypeStr=fixdt(1, 32, 30)  AccumDataTypeStr=fixdt(1, 33, 30)  SampleTime=2.5e-07
  Add1 : Sum  OutDataTypeStr=fixdt(1, 32, 30)  AccumDataTypeStr=fixdt(1, 33, 30)  SampleTime=2.5e-07
  Add2 : Sum  Inputs=+-  OutDataTypeStr=fixdt(1, 32, 30)  AccumDataTypeStr=fixdt(1, 33, 30)  SampleTime=2.5e-07
  Add3 : Sum  OutDataTypeStr=fixdt(1, 32, 30)  AccumDataTypeStr=fixdt(1, 33, 30)  SampleTime=2.5e-07
  Delay : Delay  DelayLength=double(25)  InitialCondition="fi(0,1,32,30,\"hex\",\"00000000\")"  ShowEnablePort=on
      settings: InputPortMap=u0,e6
  Delay1 : Delay  DelayLength=double(63)  InitialCondition="fi(0,1,32,30,\"hex\",\"00000000\")"  ShowEnablePort=on
      settings: InputPortMap=u0,e6
  Delay11 : Delay  DelayLength=double(70)  InitialCondition=0  SampleTime=2.5e-07
  Delay14 : Delay  DelayLength=double(1)  InitialCondition="fi(0,1,32,30,\"hex\",\"00000000\")"  ShowEnablePort=on
      settings: InputPortMap=u0,e6
  Delay2 : Delay  DelayLength=double(1)  InitialCondition="fi(0,1,32,30,\"hex\",\"00000000\")"  ShowEnablePort=on
      settings: InputPortMap=u0,e6
  Delay3 : Delay  DelayLength=double(38)  InitialCondition="fi(0,1,32,30,\"hex\",\"00000000\")"  ShowEnablePort=on
      settings: InputPortMap=u0,e6
  Delay4 : Delay  DelayLength=double(70)  InitialCondition=0  SampleTime=2.5e-07
  E1 : Outport  SampleTime=2.5e-07
  E2 : Outport  Port=2  SampleTime=2.5e-07
  wires:
  Delay1/1 -> Add2/2
  scaled1/1 -> Add/1, Delay/1
  Delay/1 -> Add/2
  validIn/1 -> Delay3/2, Delay14/2, Delay2/2, Delay1/2, Delay/2
  scaled2/1 -> Add2/1, Delay1/1
  Add/1 -> Add1/1
  Delay2/1 -> Add3/2
  Delay14/1 -> Add1/2
  Add2/1 -> Add3/1
  Add1/1 -> Delay14/1, Delay3/1
  Add3/1 -> Delay2/1, Delay4/1
  Delay3/1 -> Delay11/1
  Delay4/1 -> E2/1
  Delay11/1 -> E1/1

== system gm_soc_dvbs2_fpga/DVBS2/DVBS2 TxRx/DVB-S2 HDL Receiver/Synchronizer and PL Header Decoder/Time Frequency and Coarse Phase Synchronizer/Time and Coarse Frequency Synchronizer/Frame Synchronizer/Correlator/PLSC Correlator ==
  dataIn : Inport  OutDataTypeStr=fixdt(1, 18, 13)  PortDimensions=1  SampleTime=2.5e-07
      settings: SignalType=complex
  validIn : Inport  Port=2  OutDataTypeStr=boolean  PortDimensions=1  SampleTime=2.5e-07
  Data Type Conversion : DataTypeConversion  OutDataTypeStr=fixdt(1,18,15)  SaturateOnIntegerOverflow=off  RndMeth=Floor
  Delay : Delay  DelayLength=partlySerialExtraDelay
  Delay1 : Delay  DelayLength=partlySerialExtraDelay
  Delay3 : Delay  DelayLength=adjustDelay
  Discrete FIR Filter : dsphdlfiltering2/Discrete FIR Filter  NumeratorSource=Property  Numerator=coefs  NumeratorPrototype=[]  FilterStructure=Partly serial systolic  SerializationOption=Minimum number of cycles between valid input samples  NumCycles=shareFactor  NumberOfMultipliers=2  SimulateUsing=Code generation  roundingMode=Floor  overflowMode=off  CoefficientsDataTypeStr=Inherit: Same word length as input  OutputDataTypeStr=Inherit: Same word length as input  ResetInputPort=off  HDLGlobalReset=off  CoeffMultiplier=Multiplier  UseMultForPow2Coeff=on  FrameInputSymmOptim=off
  Discrete FIR Filter_term2 : Terminator
  Downsample : DownSample  N=shareFactor  RateOptions=Allow multirate processing
  Unit Delay Enabled Synchronous : hdlsllib/Discrete/Unit Delay Enabled Synchronous  InitialCondition=0.0  SampleTime=-1
  Upsample : dspsigops/Upsample  FactorSource=Dialog parameter  N=shareFactor  Nmax=16  phase=0  RateOptions=Allow multirate processing  ic=0  mode=Unused parameter value
  Upsample1 : dspsigops/Upsample  FactorSource=Dialog parameter  N=shareFactor  Nmax=16  phase=0  RateOptions=Allow multirate processing  ic=0  mode=Unused parameter value
  dataOut : Outport  SampleTime=2.5e-07
  wires:
  Delay/1 -> Unit Delay Enabled Synchronous/1
  dataIn/1 -> Upsample/1
  Downsample/1 -> Delay3/1
  validIn/1 -> Upsample1/1
  Discrete FIR Filter/2 -> Delay1/1
  Upsample/1 -> Discrete FIR Filter/1
  Discrete FIR Filter/3 -> Discrete FIR Filter_term2/1
  Discrete FIR Filter/1 -> Delay/1
  Upsample1/1 -> Discrete FIR Filter/2
  Delay1/1 -> Unit Delay Enabled Synchronous/2
  Unit Delay Enabled Synchronous/1 -> Downsample/1
  Delay3/1 -> Data Type Conversion/1
  Data Type Conversion/1 -> dataOut/1

== system gm_soc_dvbs2_fpga/DVBS2/DVBS2 TxRx/DVB-S2 HDL Receiver/Synchronizer and PL Header Decoder/Time Frequency and Coarse Phase Synchronizer/Time and Coarse Frequency Synchronizer/Frame Synchronizer/Correlator/SOF Correlator ==
  dataIn : Inport  OutDataTypeStr=fixdt(1, 18, 13)  PortDimensions=1  SampleTime=2.5e-07
      settings: SignalType=complex
  validIn : Inport  Port=2  OutDataTypeStr=boolean  PortDimensions=1  SampleTime=2.5e-07
  Data Type Conversion : DataTypeConversion  OutDataTypeStr=fixdt(1,18,15)  SaturateOnIntegerOverflow=off  RndMeth=Floor
  Delay : Delay  DelayLength=partlySerialExtraDelay
  Delay1 : Delay  DelayLength=partlySerialExtraDelay
  Delay3 : Delay  DelayLength=adjustDelay
  Discrete FIR Filter : dsphdlfiltering2/Discrete FIR Filter  NumeratorSource=Property  Numerator=coefs  NumeratorPrototype=[]  FilterStructure=Partly serial systolic  SerializationOption=Minimum number of cycles between valid input samples  NumCycles=shareFactor  NumberOfMultipliers=2  SimulateUsing=Code generation  roundingMode=Floor  overflowMode=off  CoefficientsDataTypeStr=Inherit: Same word length as input  OutputDataTypeStr=Inherit: Same word length as input  ResetInputPort=off  HDLGlobalReset=off  CoeffMultiplier=Multiplier  UseMultForPow2Coeff=on  FrameInputSymmOptim=off
  Discrete FIR Filter_term2 : Terminator
  Downsample : DownSample  N=shareFactor  RateOptions=Allow multirate processing
  Unit Delay Enabled Synchronous : hdlsllib/Discrete/Unit Delay Enabled Synchronous  InitialCondition=0.0  SampleTime=-1
  Upsample : dspsigops/Upsample  FactorSource=Dialog parameter  N=shareFactor  Nmax=16  phase=0  RateOptions=Allow multirate processing  ic=0  mode=Unused parameter value
  Upsample1 : dspsigops/Upsample  FactorSource=Dialog parameter  N=shareFactor  Nmax=16  phase=0  RateOptions=Allow multirate processing  ic=0  mode=Unused parameter value
  dataOut : Outport  SampleTime=2.5e-07
  wires:
  Delay/1 -> Unit Delay Enabled Synchronous/1
  dataIn/1 -> Upsample/1
  validIn/1 -> Upsample1/1
  Delay1/1 -> Unit Delay Enabled Synchronous/2
  Discrete FIR Filter/2 -> Delay1/1
  Upsample/1 -> Discrete FIR Filter/1
  Discrete FIR Filter/3 -> Discrete FIR Filter_term2/1
  Discrete FIR Filter/1 -> Delay/1
  Upsample1/1 -> Discrete FIR Filter/2
  Unit Delay Enabled Synchronous/1 -> Downsample/1
  Downsample/1 -> Delay3/1
  Delay3/1 -> Data Type Conversion/1
  Data Type Conversion/1 -> dataOut/1

== system gm_soc_dvbs2_fpga/DVBS2/DVBS2 TxRx/DVB-S2 HDL Receiver/Synchronizer and PL Header Decoder/Time Frequency and Coarse Phase Synchronizer/Time and Coarse Frequency Synchronizer/Frame Synchronizer/Pilot and Sync Pulse Indicator/ThresholdLimiter ==
  x : Inport  OutDataTypeStr=fixdt(1, 15, 12)  PortDimensions=1  SampleTime=2.5e-07
  ThresholdLimiter : MATLAB Function  TreatAsAtomicUnit=on
  y : Outport  SampleTime=2.5e-07  VectorParamsAs1DForOutWhenUnconnected=off
  wires:
  ThresholdLimiter/1(y) -> y/1
  x/1 -> ThresholdLimiter/1(x)

== system gm_soc_dvbs2_fpga/DVBS2/DVBS2 TxRx/DVB-S2 HDL Receiver/Synchronizer and PL Header Decoder/Time Frequency and Coarse Phase Synchronizer/Time and Coarse Frequency Synchronizer/PL Data Descrambler and Pilot Valid Indicator/PL Data Descrambler/PL Scramble Sequence Mapper LUT ==
  In1 : Inport
  PL Scramble Sequence Mapper LUT : Lookup_n-D  NumberOfTableDimensions=1  LookupTableObject=''  BreakpointsSpecification=Even spacing  BreakpointsForDimension1=[-5:5]  BreakpointsForDimension1FirstPoint=0  BreakpointsForDimension2FirstPoint=10  BreakpointsForDimension2Spacing=12  IndexSearchMethod=Evenly spaced points  Table=[1;1i;-1;-1i]  TableDataTypeStr=fixdt(1,2,0)  InterpMethod=Flat  InternalRulePriority=Speed  OutDataTypeStr=fixdt(1,2,0)  RndMeth=Simplest
  PL Scramble Sequence Mapper LUT_pd1 : Delay  DelayLength=1
  Out1 : Outport
  wires:
  In1/1 -> PL Scramble Sequence Mapper LUT/1
  PL Scramble Sequence Mapper LUT_pd1/1 -> Out1/1
  PL Scramble Sequence Mapper LUT/1 -> PL Scramble Sequence Mapper LUT_pd1/1

== system gm_soc_dvbs2_fpga/DVBS2/DVBS2 TxRx/DVB-S2 HDL Receiver/Synchronizer and PL Header Decoder/Time Frequency and Coarse Phase Synchronizer/Time and Coarse Frequency Synchronizer/PL Data Descrambler and Pilot Valid Indicator/PL Data Descrambler/PL Scrambler Gold Sequence Generator ==
  reset : Inport  OutDataTypeStr=boolean  PortDimensions=1  SampleTime=2.5e-07
  validIn : Inport  Port=2  OutDataTypeStr=boolean  PortDimensions=1  SampleTime=2.5e-07
  Bit Concat : hdlsllib/Logic and Bit Operations/Bit Concat  numInputs=2
  Delay{,3..4,10,12..15} (8 alike) : Delay  DelayLength=1
  Delay{1..2,5..9,11} (8 alike) : Delay
  Logical Operator : Logic  Operator=XOR  AllPortsSameDT=off  OutDataTypeStr=boolean
  Logical Operator1 : Logic  Operator=XOR  AllPortsSameDT=off  OutDataTypeStr=boolean
  Logical Operator2 : Logic  Operator=OR  AllPortsSameDT=off  OutDataTypeStr=boolean
  Subsystem : Subsystem
  dataOut : Outport  SampleTime=2.5e-07
  validOut : Outport  Port=2  SampleTime=2.5e-07
  wires:
  reset/1 -> Delay3/1
  Subsystem/1(xMnp131072) -> Delay6/1
  validIn/1 -> Delay4/1
  Delay5/1 -> Delay13/1
  Delay13/1 -> Delay15/1
  Delay/1 -> Delay11/1, Logical Operator2/2
  Delay3/1 -> Delay/1
  Delay2/1 -> Delay5/1
  Delay4/1 -> Logical Operator2/1, Delay2/1
  Logical Operator2/1 -> Delay1/1
  Delay8/1 -> Logical Operator/1
  Delay1/1 -> Subsystem/Enable
  Delay11/1 -> Subsystem/1(reset)
  Subsystem/2(yM131072) -> Delay7/1
  Subsystem/3(xMn) -> Delay8/1
  Subsystem/4(yM0) -> Delay9/1
  Delay10/1 -> Bit Concat/1
  Delay15/1 -> validOut/1
  Delay6/1 -> Logical Operator1/1
  Delay7/1 -> Logical Operator1/2
  Delay9/1 -> Logical Operator/2
  Logical Operator1/1 -> Delay10/1
  Logical Operator/1 -> Delay12/1
  Delay12/1 -> Bit Concat/2
  Bit Concat/1 -> Delay14/1
  Delay14/1 -> dataOut/1

== system gm_soc_dvbs2_fpga/DVBS2/DVBS2 TxRx/DVB-S2 HDL Receiver/Synchronizer and PL Header Decoder/Time Frequency and Coarse Phase Synchronizer/Time and Coarse Frequency Synchronizer/Symbol Synchronizer/Gardner TED/GTED ==
  In1 : Inport  OutDataTypeStr=fixdt(1, 22, 13)  PortDimensions=1  SampleTime=6.25e-08
      settings: SignalType=complex
  Add : Sum  OutDataTypeStr=fixdt(1, 46, 26)
  Add1 : Sum  Inputs=+-  OutDataTypeStr=fixdt(1, 23, 13)
  Add2 : Sum  Inputs=+-  OutDataTypeStr=fixdt(1, 23, 13)
  Complex to Real-Imag : ComplexToRealImag
  Delay{,1..7} (8 alike) : Delay  DelayLength=1
  Delay{8..13} (6 alike) : Delay
  Product : Product  OutDataTypeStr=fixdt(1, 45, 26)
  Product1 : Product  OutDataTypeStr=fixdt(1, 45, 26)
  Out1 : Outport  SampleTime=6.25e-08
  wires:
  In1/1 -> Complex to Real-Imag/1
  Complex to Real-Imag/1 -> Add1/2, Delay/1
  Complex to Real-Imag/2 -> Add2/2, Delay4/1
  Delay2/1 -> Delay3/1
  Delay4/1 -> Delay5/1
  Delay/1 -> Delay1/1
  Product/1 -> Delay10/1
  Add2/1 -> Delay12/1
  Delay5/1 -> Delay11/1, Delay6/1
  Add/1 -> Out1/1
  Delay1/1 -> Delay8/1, Delay2/1
  Delay6/1 -> Delay7/1
  Delay8/1 -> Product/1
  Delay3/1 -> Add1/1
  Delay7/1 -> Add2/1
  Delay9/1 -> Product/2
  Add1/1 -> Delay9/1
  Delay11/1 -> Product1/1
  Delay12/1 -> Product1/2
  Delay13/1 -> Add/2
  Product1/1 -> Delay13/1
  Delay10/1 -> Add/1

== system gm_soc_dvbs2_fpga/DVBS2/DVBS2 TxRx/DVB-S2 HDL Receiver/Synchronizer and PL Header Decoder/Time Frequency and Coarse Phase Synchronizer/Time and Coarse Frequency Synchronizer/Symbol Synchronizer/Rate Handle/FIFO ==
  data : Inport  OutDataTypeStr=fixdt(1, 18, 13)  PortDimensions=1  SampleTime=6.25e-08
      settings: SignalType=complex
  push : Inport  Port=2  OutDataTypeStr=boolean  PortDimensions=1  SampleTime=6.25e-08
  pop : Inport  Port=3  OutDataTypeStr=boolean  PortDimensions=1  SampleTime=6.25e-08
  Delay1 : Delay  DelayLength=double(1)  InitialCondition=0  SampleTime=6.25e-08
  Delay2 : Delay  DelayLength=double(1)  InitialCondition=0  SampleTime=6.25e-08
  HDL Counter : hdlsllib/Sources/HDL Counter  CountType=Count limited  CountInit=0  CountStep=1  CountMax=1024-1  CountFromType=Initial value  CountFrom=0  CountResetPort=off  CountLoadPort=off  CountEnbPort=on  CountDirPort=off  CountHitOutputPort=off  CountDataType=Unsigned  CountWordLen=nextpow2(1024-1)  CountFracLen=0  CountSampTime=1
  HDL Counter1 : hdlsllib/Sources/HDL Counter  CountType=Count limited  CountInit=0  CountStep=1  CountMax=1024 - 1  CountFromType=Initial value  CountFrom=0  CountResetPort=off  CountLoadPort=off  CountEnbPort=on  CountDirPort=off  CountHitOutputPort=off  CountDataType=Unsigned  CountWordLen=nextpow2(1024-1)  CountFracLen=0  CountSampTime=1
  Logical Operator : Logic  AllPortsSameDT=off  OutDataTypeStr=boolean  SampleTime=6.25e-08
  Logical Operator1 : Logic  Operator=OR  AllPortsSameDT=off  OutDataTypeStr=boolean  SampleTime=6.25e-08
  Logical Operator2 : Logic  Operator=NOT  Inputs=1  AllPortsSameDT=off  OutDataTypeStr=boolean  SampleTime=6.25e-08
  Logical Operator3 : Logic  AllPortsSameDT=off  OutDataTypeStr=boolean  SampleTime=6.25e-08
  MATLAB Function : Subsystem
  Simple Dual Port RAM : hdlsllib/HDL RAMs/Simple Dual Port RAM  ram_size=nextpow2(1024-1)
  out : Outport  SampleTime=6.25e-08
  outValid : Outport  Port=2  SampleTime=6.25e-08
  wires:
  Logical Operator3/1 -> MATLAB Function/2(rd), Logical Operator1/2, outValid/1
  Logical Operator2/1 -> Logical Operator3/1
  Delay2/1 -> Logical Operator2/1
  HDL Counter/1 -> Simple Dual Port RAM/2
  push/1 -> Logical Operator/1, HDL Counter/1, MATLAB Function/1(wr), Simple Dual Port RAM/3
  Logical Operator/1 -> Logical Operator1/1
  MATLAB Function/1(full) -> Delay1/1
  MATLAB Function/2(empty) -> Delay2/1
  pop/1 -> Logical Operator3/2
  data/1 -> Simple Dual Port RAM/1
  Delay1/1 -> Logical Operator/2
  Logical Operator1/1 -> HDL Counter1/1
  HDL Counter1/1 -> Simple Dual Port RAM/4
  Simple Dual Port RAM/1 -> out/1

== system gm_soc_dvbs2_fpga/DVBS2/DVBS2 TxRx/DVB-S2 HDL Receiver/Synchronizer and PL Header Decoder/Time Frequency and Coarse Phase Synchronizer/Time and Coarse Frequency Synchronizer/Symbol Synchronizer/Rate Handle/monostable ==
  trigger : Inport  OutDataTypeStr=boolean  PortDimensions=1  SampleTime=6.25e-08
  monostable : MATLAB Function  TreatAsAtomicUnit=on  mask{nClocks=config.SamplesPerSymbol}
      mask prompts: nClocks "Number of Clocks:"
  out : Outport  SampleTime=6.25e-08  VectorParamsAs1DForOutWhenUnconnected=off
  wires:
  trigger/1 -> monostable/1(trigger)
  monostable/1(out) -> out/1
